simulink subsystem "voltage_to_kelvin_subsystem"  (R2020b)
settings: Solver=VariableStepAuto  StartTime=0.0  StopTime=10.0  RelTol=1e-3
settings Model: Creator=Milind  LastModifiedBy=Milind

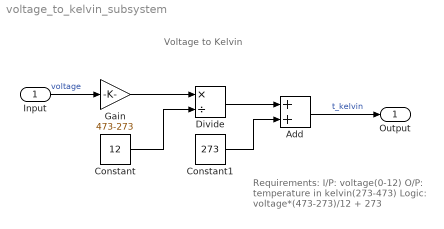
== system voltage_to_kelvin_subsystem ==
  note: Requirements:
      | I/P: voltage(0-12)
      | O/P: temperature in kelvin(273-473)
      | Logic: voltage*(473-273)/12 + 273
  note: Voltage to Kelvin
  Input : Inport
  Add : Sum
  Constant : Constant  Value=12
  Constant1 : Constant  Value=273
  Divide : Product  Inputs=*/
  Gain : Gain  Gain=473-273
  Output : Outport
  wires:
  Constant/1 -> Divide/2
  Input/1 -> Gain/1  "voltage"
  Add/1 -> Output/1  "t_kelvin"
  Constant1/1 -> Add/2
  Gain/1 -> Divide/1
  Divide/1 -> Add/1
